simulink model "untitled"  (R2014b)
settings: Solver=ode45  StartTime=0.0  StopTime=50.0  RelTol=1e-3
undefined symbols (not defined in the file): k0, s1, s2, sigbuilder_block, td, ti
settings Model: Creator=root  LastModifiedBy=root

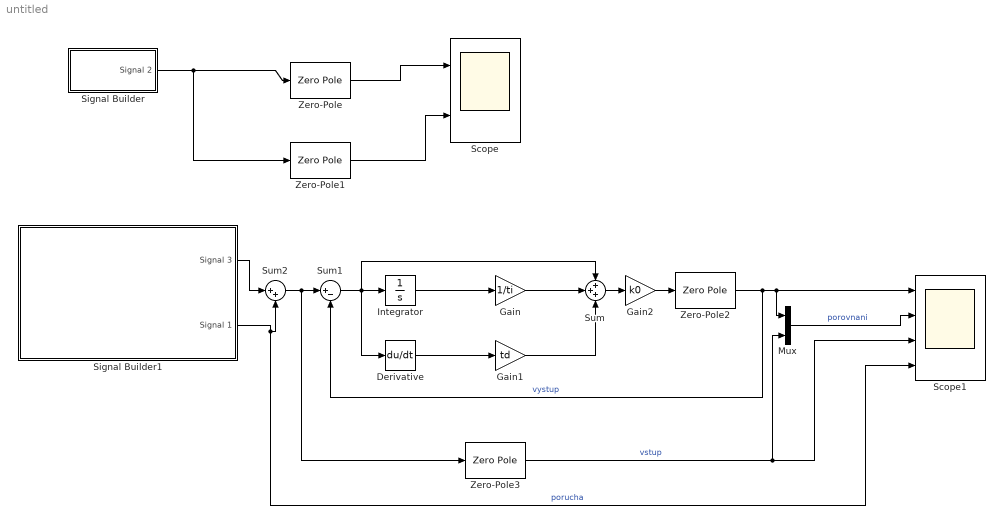
== system untitled ==
  Derivative : Derivative
  Gain : Gain  Gain=1/ti
  Gain1 : Gain  Gain=td
  Gain2 : Gain  Gain=k0
  Integrator : Integrator
  Mux : Mux  Inputs=2
  Scope : Scope  NumInputPorts=2
      settings: YMin=-1~-1  YMax=1~1
  Scope1 : Scope  NumInputPorts=4
      settings: YMin=-1~-5~-5~-5  YMax=1~5~5~5
  Signal Builder : Subsystem  Tag=STV Subsys  LoadFcn=sigbuilder_block('load');  StartFcn=sigbuilder_block('start');  StopFcn=sigbuilder_block('stop');  ClipboardFcn=sigbuilder_block('clipboard');  mask(Sigbuilder block){}
      mask help: Simulink:masks:SigbuilderBlock_MD
      mask init:
      | if ~strcmp(get_param(bdroot(gcbh),'SimulationStatus'),'stopped') tuvar = sigbuilder_block('maskInit'); end
      settings: CopyFcn=sigbuilder_block('copy');  DeleteFcn=sigbuilder_block('delete');  ModelCloseFcn=sigbuilder_block('modelClose');  PreSaveFcn=sigbuilder_block('preSave');  PauseFcn=sigbuilder_block('pause');  ContinueFcn=sigbuilder_block('continue');  NameChangeFcn=sigbuilder_block('namechange');  OpenFcn=sigbuilder_block('open',[437.6 199.2 550.4 400 ]);  CloseFcn=sigbuilder_block('close');
      mask Display: plot(0, 0, 100, 100,[2, 2, 32, 32, 2], [68, 8, 8, 68, 68],[32, 2], [38, 38], [32, 19, 2],[53, 60, 44], [32, 17, 17, 2],[16, 16, 31, 31]);txt = getActiveGroup(gcbh);text(2, 100, txt,'verticalAlignment', 'top');
  Signal Builder1 : Subsystem  Tag=STV Subsys  LoadFcn=sigbuilder_block('load');  StartFcn=sigbuilder_block('start');  StopFcn=sigbuilder_block('stop');  ClipboardFcn=sigbuilder_block('clipboard');  mask(Sigbuilder block){}
      mask help: Simulink:masks:SigbuilderBlock_MD
      mask init:
      | if ~strcmp(get_param(bdroot(gcbh),'SimulationStatus'),'stopped') tuvar = sigbuilder_block('maskInit'); end
      settings: CopyFcn=sigbuilder_block('copy');  DeleteFcn=sigbuilder_block('delete');  ModelCloseFcn=sigbuilder_block('modelClose');  PreSaveFcn=sigbuilder_block('preSave');  PauseFcn=sigbuilder_block('pause');  ContinueFcn=sigbuilder_block('continue');  NameChangeFcn=sigbuilder_block('namechange');  OpenFcn=sigbuilder_block('open',[437.6 199.2 550.4 400 ]);  CloseFcn=sigbuilder_block('close');
      mask Display: plot(0, 0, 100, 100,[2, 2, 32, 32, 2], [68, 8, 8, 68, 68],[32, 2], [38, 38], [32, 19, 2],[53, 60, 44], [32, 17, 17, 2],[16, 16, 31, 31]);txt = getActiveGroup(gcbh);text(2, 100, txt,'verticalAlignment', 'top');
  Sum : Sum  Inputs=+++
  Sum1 : Sum  Inputs=|+-
  Sum2 : Sum  Inputs=|++
  Zero-Pole : ZeroPole  Zeros=[]  Poles=[s1 s2]
  Zero-Pole1 : ZeroPole  Zeros=[]  Poles=[s1 s2]  Gain=[abs(s1*s2)]
  Zero-Pole2 : ZeroPole  Zeros=[]  Poles=[s1 s2]
  Zero-Pole3 : ZeroPole  Zeros=[]  Poles=[s1 s2]
  wires:
  Signal Builder/1(Signal 2) -> Zero-Pole1/1, Zero-Pole/1
  Zero-Pole/1 -> Scope/1
  Zero-Pole1/1 -> Scope/2
  Integrator/1 -> Gain/1
  Derivative/1 -> Gain1/1
  Gain/1 -> Sum/2
  Gain1/1 -> Sum/3
  Sum/1 -> Gain2/1
  Zero-Pole2/1 -> Sum1/2, Mux/1, Scope1/1  "vystup"
  Sum1/1 -> Sum/1, Integrator/1, Derivative/1
  Gain2/1 -> Zero-Pole2/1
  Zero-Pole3/1 -> Mux/2, Scope1/3  "vstup"
  Mux/1 -> Scope1/2  "porovnani"
  Signal Builder1/2(Signal 1) -> Sum2/2, Scope1/4  "porucha"
  Sum2/1 -> Zero-Pole3/1, Sum1/1
  Signal Builder1/1(Signal 3) -> Sum2/1

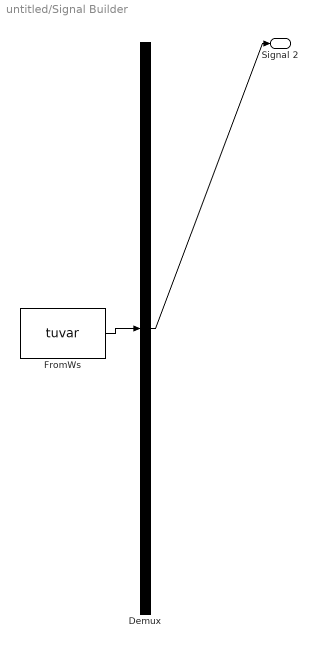
== system untitled/Signal Builder ==
  Demux : Demux  Tag=STV Demux  Outputs=1
  FromWs : FromWorkspace  Tag=STV FromWs  VariableName=tuvar  SampleTime=0
      SigBuilderData=|
      | common.afterFinalStr = 'Extrapolate'
      | common.sampleTime = 0
      | dataSet.timeRange = [0 10]
      | dataSet.name = 'Group 1'
      | sbobj.Groups.Name = 'Group 1'
      | sbobj.Groups.Signals.Name = 'Signal 2'
      | sbobj.Groups.Signals.XData = [0 5 5 10]
      | sbobj.Groups.Signals.YData = [0 0 1 1]
  Signal 2 : Outport  Tag=STV Outport
  wires:
  FromWs/1 -> Demux/1
  Demux/1 -> Signal 2/1

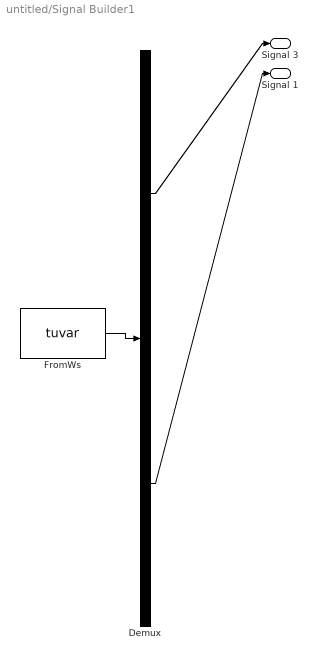
== system untitled/Signal Builder1 ==
  Demux : Demux  Tag=STV Demux  Outputs=2
  FromWs : FromWorkspace  Tag=STV FromWs  VariableName=tuvar  SampleTime=0
      SigBuilderData=|
      | common.afterFinalStr = 'Extrapolate'
      | common.sampleTime = 0
      | dataSet.timeRange = [0 24]
      | dataSet.name = 'Group 1'
      | sbobj.Groups.Name = 'Group 1'
      | sbobj.Groups.Signals(1).Name = 'Signal 3'
      | sbobj.Groups.Signals(1).XData = [0 5 5 23 23 24]
      | sbobj.Groups.Signals(1).YData = [19 19 23 23 19 19]
      | sbobj.Groups.Signals(2).Name = 'Signal 1'
      | sbobj.Groups.Signals(2).XData = [0 14 14 18 18 24]
      | sbobj.Groups.Signals(2).YData = [0 0 -3 -3 0 0]
      | sbobj.Groups.TimeRange = [0 24]
  Signal 3 : Outport  Tag=STV Outport
  Signal 1 : Outport  Tag=STV Outport  Port=2
  wires:
  FromWs/1 -> Demux/1
  Demux/1 -> Signal 3/1
  Demux/2 -> Signal 1/1
